simulink model "CF016A_GmVehSpdArbn"  (R2013b)
settings: Solver=FixedStepDiscrete  SolverMode=SingleTasking  StartTime=0.0  StopTime=1  FixedStep=0.002  RelTol=1e-3
undefined symbols (not defined in the file): DIAGCSTRTUPDLY_CNT_U32, NODEBSTEP_CNT_U16, NtcNr1, NtcSts1, VEHSPDMAX_KPH_F32
libraries: simulink x8, NxtrMax x7, NxtrMin x3, NxtrLim x3
(part 1 of 5)
settings Model: PauseTimes=2  CovMetricSettings=dcmrw  CovFilter=CF09_GMOverlayStateHandler_v002_covfilter  CovHTMLOptions=-sRT=1 -aTS=1 -bRG=1 -bTC=1 -hTR=0 -nFC=0 -scm=1 -bcm=1 -xEv=0  covSaveCumulativeToWorkspaceVar=off  CovSaveSingleToWorkspaceVar=off  CovCumulativeReport=on  Creator=SZ7VY6  LastModifiedBy=sz7vy6
settings SolverCC: AutoInsertRateTranBlk=on  InsertRTBMode=Always
settings DataIOCC: LimitDataPoints=off  SaveFormat=Structure  ReturnWorkspaceOutputs=on
settings OptimizationCC: BlockReduction=off  InlineParams=on  ZeroExternalMemoryAtStartup=off  ZeroInternalMemoryAtStartup=off  OptimizeModelRefInitCode=on  LifeSpan=1
settings DebuggingCC: SignalInfNanChecking=error  SignalRangeChecking=warning  UnderspecifiedInitializationDetection=Simplified  SolverPrmCheckMsg=error  InheritedTsInSrcMsg=error  DiscreteInheritContinuousMsg=error  SingleTaskRateTransMsg=error  TasksWithSamePriorityMsg=error  SigSpecEnsureSampleTimeMsg=error  CheckMatrixSingularityMsg=error  ParameterUnderflowMsg=error  ParameterPrecisionLossMsg=error  ParameterTunabilityLossMsg=error  FixptConstUnderflowMsg=warning  FixptConstOverflowMsg=warning  VectorMatrixConversionMsg=error  SignalLabelMismatchMsg=error  UnconnectedInputMsg=error  UnconnectedOutputMsg=error  UnconnectedLineMsg=error  SFcnCompatibilityMsg=error  UniqueDataStoreMsg=warning  BusObjectLabelMismatch=error  RootOutportRequireBusObject=error  AssertControl=DisableAll  ModelReferenceIOMsg=error  ModelReferenceVersionMismatchMessage=warning  ModelReferenceIOMismatchMessage=error  ModelReferenceCSMismatchMessage=warning  ModelReferenceDataLoggingMessage=error  StateNameClashWarn=warning  StrictBusMsg=ErrorOnBusTreatedAsVector  NonBusSignalsTreatedAsBus=error  SFUnexpectedBacktrackingDiag=error  SFInvalidInputDataAccessInChartInitDiag=error  SFNoUnconditionalDefaultTransitionDiag=error  SFTransitionOutsideNaturalParentDiag=error  SFUnconditionalTransitionShadowingDiag=error  SFUndirectedBroadcastEventsDiag=error
settings ModelReferenceCC: ModelReferenceNumInstancesAllowed=Single
settings RTWCC: SystemTargetFile=autosar.tlc  GenCodeOnly=on  TemplateMakefile=ert_default_tmf  Description=AUTOSAR  GenerateReport=on  ProcessScript=autosar_make_rtw_hook  LaunchReport=on
settings CodeAppCC: GenerateComments=off  IgnoreCustomStorageClasses=off  CustomSymbolStrType=$N$R$M  CustomSymbolStrBlkIO=$N$M  SimulinkBlockComments=off
settings STFCustomTargetCC: ParMdlRefBuildCompliant=on  CompOptLevelCompliant=on  IncludeMdlTerminateFcn=off  CombineOutputUpdateFcns=on  SuppressErrorStatus=on  ERTFirstTimeCompliant=on  ERTCustomFileBanners=on  SupportNonFinite=off  SupportComplex=off  SupportContinuousTime=off  SupportNonInlinedSFcns=off  MATLABClassNameForMDSCustomization=Simulink.SoftwareTarget.ERTCustomization  AutosarCompliant=on  GRTInterface=off  SystemTargetFile=autosar.tlc
settings ERTTargetCC: CodeReplacementLibrary=ANSI_C  ConcurrentExecutionCompliant=off  IncludeMdlTerminateFcn=off  SuppressErrorStatus=on  SupportNonFinite=off  SupportComplex=off  ModelStepFunctionPrototypeControlCompliant=off  CPPClassGenCompliant=off  AutosarCompliant=on  InlinedParameterPlacement=NonHierarchical  ERTCustomFileTemplate=example_file_process.tlc  EnableUserReplacementTypes=on

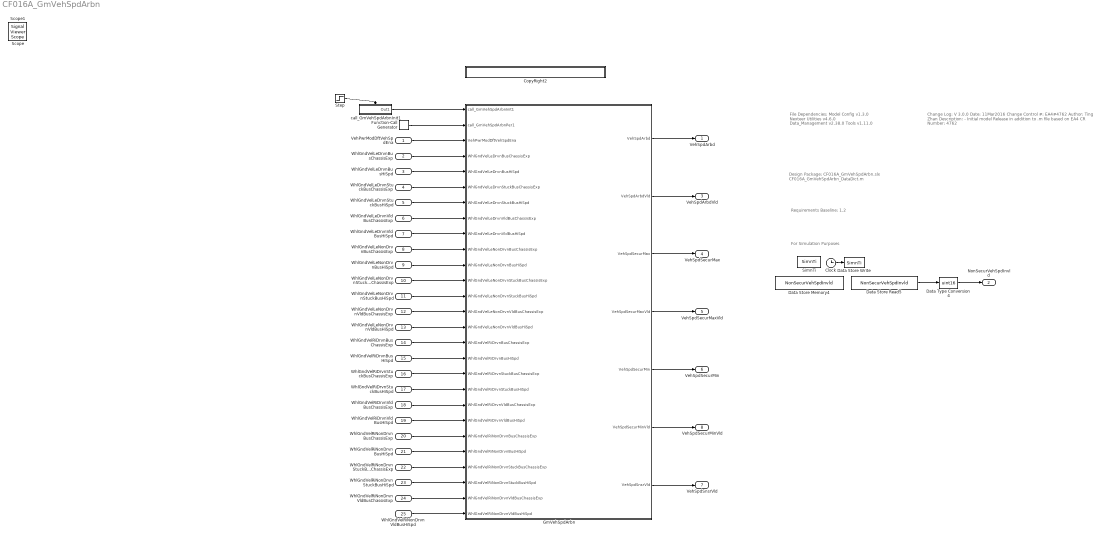
== system CF016A_GmVehSpdArbn ==
  note: File Dependencies:
      |
      | Model Config v1.3.0
      | Nexteer Utilities v4.6.0
      | Data_Management v2.38.0
      | Tools v1.11.0
  note: Requirements Baseline: 1.2
  note: Change Log:
      |
      | V 3.0.0
      | Date: 11Mar2016
      | Change Control #: EA4#4762
      | Author: Ting Zhan
      | Description:
      | - Initial model Release in addition to .m file based on EA4
      | CR Number: 4762
  note: For Simulation Purposes
  note: Design Package:
      | CF016A_GmVehSpdArbn.slx
      | CF016A_GmVehSpdArbn_DataDict.m
  VehPwrModDftVehSpdEna : Inport  RequirementInfo={} %GIDa_1b9c6812_2c02_4b85_9a2c_669458cc48bb  OutDataTypeStr=boolean
  WhlGndVelLeDrvnBusChassisExp : Inport  RequirementInfo={} %GIDa_f6a8d43a_8d7a_4621_b19c_bbf61fc3f1fb  Port=2  OutDataTypeStr=single
  WhlGndVelLeDrvnBusHiSpd : Inport  RequirementInfo={} %GIDa_8d06928a_e9dc_4bb5_bb38_60b41e7e1a37  Port=3  OutDataTypeStr=single
  WhlGndVelLeDrvnStuckBusChassisExp : Inport  RequirementInfo={} %GIDa_37f18a4c_7dd2_4559_8edf_851675215370  Port=4  OutDataTypeStr=boolean
  WhlGndVelLeDrvnStuckBusHiSpd : Inport  RequirementInfo={} %GIDa_387e051a_cae3_4bd1_96b6_4bb2f8da8f18  Port=5  OutDataTypeStr=boolean
  WhlGndVelLeDrvnVldBusChassisExp : Inport  RequirementInfo={} %GIDa_835686fb_41df_4b3b_981b_1312eb084a3e  Port=6  OutDataTypeStr=boolean
  WhlGndVelLeDrvnVldBusHiSpd : Inport  RequirementInfo={} %GIDa_951897dd_207e_4223_8bb8_db091924bf4f  Port=7  OutDataTypeStr=boolean
  WhlGndVelLeNonDrvnBusChassisExp : Inport  RequirementInfo={} %GIDa_a4eac490_54c7_4771_95de_17d76ce0ec27  Port=8  OutDataTypeStr=single
  WhlGndVelLeNonDrvnBusHiSpd : Inport  RequirementInfo={} %GIDa_08a6082e_b874_4a55_b94e_1af7c22679ef  Port=9  OutDataTypeStr=single
  WhlGndVelLeNonDrvnStuckBusChassisExp : Inport  RequirementInfo={} %GIDa_8ce78da2_9eb9_457c_9700_f53d3d0bd86d  Port=10  OutDataTypeStr=boolean
  WhlGndVelLeNonDrvnStuckBusHiSpd : Inport  RequirementInfo={} %GIDa_514e7ca7_7671_44d6_bb21_5a584f285d08  Port=11  OutDataTypeStr=boolean
  WhlGndVelLeNonDrvnVldBusChassisExp : Inport  RequirementInfo={} %GIDa_350e08e4_76f4_4ea8_8a72_cd9a2d5bb9fc  Port=12  OutDataTypeStr=boolean
  WhlGndVelLeNonDrvnVldBusHiSpd : Inport  RequirementInfo={} %GIDa_e452ab69_b19c_414f_baf2_b1cca5193dc7  Port=13  OutDataTypeStr=boolean
  WhlGndVelRiDrvnBusChassisExp : Inport  RequirementInfo={} %GIDa_febb2255_174e_400c_a750_3a2634fb8d82  Port=14  OutDataTypeStr=single
  WhlGndVelRiDrvnBusHiSpd : Inport  RequirementInfo={} %GIDa_33e5a17e_e6ff_4c9b_8e04_aa687b674ac0  Port=15  OutDataTypeStr=single
  WhlGndVelRiDrvnStuckBusChassisExp : Inport  RequirementInfo={} %GIDa_eb4592a4_6e28_4790_a7e9_7dfcd52d8359  Port=16  OutDataTypeStr=boolean
  WhlGndVelRiDrvnStuckBusHiSpd : Inport  RequirementInfo={} %GIDa_4d5fec21_2deb_48fd_8ba8_4b270e8dc755  Port=17  OutDataTypeStr=boolean
  WhlGndVelRiDrvnVldBusChassisExp : Inport  RequirementInfo={} %GIDa_0045e6f2_b2f6_4af3_8c4b_d2a93e5e542f  Port=18  OutDataTypeStr=boolean
  WhlGndVelRiDrvnVldBusHiSpd : Inport  RequirementInfo={} %GIDa_aa92ccdb_2b03_48a5_9a02_c9af57aaf9ac  Port=19  OutDataTypeStr=boolean
  WhlGndVelRiNonDrvnBusChassisExp : Inport  RequirementInfo={} %GIDa_6a49e4d8_e7ef_45b6_ac02_9148e779a1b3  Port=20  OutDataTypeStr=single
  WhlGndVelRiNonDrvnBusHiSpd : Inport  RequirementInfo={} %GIDa_c3dbff61_00f7_4638_9308_f36d29dc0e51  Port=21  OutDataTypeStr=single
  WhlGndVelRiNonDrvnStuckBusChassisExp : Inport  RequirementInfo={} %GIDa_d960e54b_b41b_4df2_9791_080f8c78f146  Port=22  OutDataTypeStr=boolean
  WhlGndVelRiNonDrvnStuckBusHiSpd : Inport  RequirementInfo={} %GIDa_679668c6_3c13_4074_8295_9c18477c1537  Port=23  OutDataTypeStr=boolean
  WhlGndVelRiNonDrvnVldBusChassisExp : Inport  RequirementInfo={} %GIDa_7aefde58_d94c_4a0b_882a_fddc487b4430  Port=24  OutDataTypeStr=boolean
  WhlGndVelRiNonDrvnVldBusHiSpd : Inport  RequirementInfo={} %GIDa_14985695_b713_4ff3_87b9_d780a2a8766e  Port=25  OutDataTypeStr=boolean
  Clock : Clock
  CopyRight2 : Subsystem  Description=|  mask(Copyright Information){none=on}
      | Copyright info block.                                               
      |                                                                     
      | Place copyright information at the top of every subsystem in design.
      mask prompts: none "No parameters"
      mask help: Place copyright information at the top of every subsystem in design.
      mask Display:
      | NxtrConf = 'Nexteer Confidential';
      | 
      | sys = bdroot; %handle for the current model ("system")
      | first = get_param(sys,'Created');
      | if(isempty(first))
      |     first = datestr(now,'yyyy');
      | else
      |     first = first(end-3:end);  %year is last four digits
      | end
      | 
      | last = get_param(sys,'LastModifiedDate');
      | if isempty(last)
      |     last = datestr(now,'yyyy');
      | else
      |     last = last(end-3:end);
      | end
      | 
      | if strcmp(first,last)
      |     fprintf('%s -- Copyright %s Nexteer',NxtrConf,first)
      | else
      |     fprintf('%s -- %s%s- %s Nexteer',NxtrConf,char(169),first,last)
      | end
  Data Store Memory4 : DataStoreMemory  DataStoreName=NonSecurVehSpdInvld  InitialValue=NtcSts1.NTCSTS_PASSD  OutDataTypeStr=Enum: NtcSts1
  Data Store Read5 : DataStoreRead  DataStoreName=NonSecurVehSpdInvld  SampleTime=.004
  Data Store Write : DataStoreWrite  DataStoreName=SimnTi
  Data Type Conversion4 : DataTypeConversion  OutDataTypeStr=uint16
  Function-Call Generator : simulink/Ports & Subsystems/Function-Call Generator  sample_time=.01  numberOfIterations=1
      settings: AttributesFormatString=%<sample_time>
  GmVehSpdArbn : Subsystem  RequirementInfo="{}  %GIDa_c04c64db_09f4_4bf6_ae81_75ae0555dc21"
  SimnTi : DataStoreMemory  DataStoreName=SimnTi
  Step : Step  Time=.001  Before=1  After=0  SampleTime=0
  call_GmVehSpdArbnInit1 : Subsystem  TreatAsAtomicUnit=on
  VehSpdArbd : Outport  RequirementInfo={} %GIDa_1da87020_2114_47f8_bd6a_dcf122c70ef9
  NonSecurVehSpdInvld : Outport  RequirementInfo={} %GIDa_f8f24313_b0b7_4842_bede_f0c570d36cae  Port=2
  VehSpdArbdVld : Outport  RequirementInfo={} %GIDa_aeae8495_df44_455f_bfcb_3785565b89f3  Port=3
  VehSpdSecurMax : Outport  RequirementInfo={} %GIDa_e60aac24_3e4f_4fa4_92d1_30c110927cae  Port=4
  VehSpdSecurMaxVld : Outport  RequirementInfo={} %GIDa_e0614fd2_7d45_427f_a7be_e9487d2cc3f6  Port=5
  VehSpdSecurMin : Outport  RequirementInfo={} %GIDa_5226fce9_09b3_4eff_a0f8_954e16115eec  Port=6
  VehSpdSnsrVld : Outport  RequirementInfo={} %GIDa_37fde451_082a_4d0c_b5e1_d1c1d8bf7c50  Port=7
  VehSpdSecurMinVld : Outport  RequirementInfo={} %GIDa_3de6a7fd_89af_4cb9_baa0_fb7c34e7cace  Port=8
  Scope : SignalViewerScope  IOType=viewer  RefreshTime=0.035000
  Scope1 : SignalViewerScope  IOType=viewer  RefreshTime=0.035000
  wires:
  Step/1 -> call_GmVehSpdArbnInit1/Enable
  call_GmVehSpdArbnInit1/1(Out1) -> GmVehSpdArbn/1(call_GmVehSpdArbnInit1)
  Clock/1 -> Data Store Write/1
  GmVehSpdArbn/1(VehSpdArbd) -> VehSpdArbd/1
  Data Store Read5/1 -> Data Type Conversion4/1
  Data Type Conversion4/1 -> NonSecurVehSpdInvld/1
  Function-Call Generator/1 -> GmVehSpdArbn/2(call_GmVehSpdArbnPer1)
  VehPwrModDftVehSpdEna/1 -> GmVehSpdArbn/3(VehPwrModDftVehSpdEna)
  WhlGndVelLeDrvnBusChassisExp/1 -> GmVehSpdArbn/4(WhlGndVelLeDrvnBusChassisExp)
  WhlGndVelLeDrvnBusHiSpd/1 -> GmVehSpdArbn/5(WhlGndVelLeDrvnBusHiSpd)
  WhlGndVelLeDrvnStuckBusChassisExp/1 -> GmVehSpdArbn/6(WhlGndVelLeDrvnStuckBusChassisExp)
  WhlGndVelLeDrvnStuckBusHiSpd/1 -> GmVehSpdArbn/7(WhlGndVelLeDrvnStuckBusHiSpd)
  WhlGndVelLeDrvnVldBusChassisExp/1 -> GmVehSpdArbn/8(WhlGndVelLeDrvnVldBusChassisExp)
  WhlGndVelLeDrvnVldBusHiSpd/1 -> GmVehSpdArbn/9(WhlGndVelLeDrvnVldBusHiSpd)
  WhlGndVelLeNonDrvnBusChassisExp/1 -> GmVehSpdArbn/10(WhlGndVelLeNonDrvnBusChassisExp)
  WhlGndVelLeNonDrvnBusHiSpd/1 -> GmVehSpdArbn/11(WhlGndVelLeNonDrvnBusHiSpd)
  WhlGndVelLeNonDrvnStuckBusChassisExp/1 -> GmVehSpdArbn/12(WhlGndVelLeNonDrvnStuckBusChassisExp)
  WhlGndVelLeNonDrvnStuckBusHiSpd/1 -> GmVehSpdArbn/13(WhlGndVelLeNonDrvnStuckBusHiSpd)
  WhlGndVelLeNonDrvnVldBusChassisExp/1 -> GmVehSpdArbn/14(WhlGndVelLeNonDrvnVldBusChassisExp)
  WhlGndVelLeNonDrvnVldBusHiSpd/1 -> GmVehSpdArbn/15(WhlGndVelLeNonDrvnVldBusHiSpd)
  WhlGndVelRiDrvnBusChassisExp/1 -> GmVehSpdArbn/16(WhlGndVelRiDrvnBusChassisExp)
  WhlGndVelRiDrvnBusHiSpd/1 -> GmVehSpdArbn/17(WhlGndVelRiDrvnBusHiSpd)
  WhlGndVelRiDrvnStuckBusChassisExp/1 -> GmVehSpdArbn/18(WhlGndVelRiDrvnStuckBusChassisExp)
  WhlGndVelRiDrvnStuckBusHiSpd/1 -> GmVehSpdArbn/19(WhlGndVelRiDrvnStuckBusHiSpd)
  WhlGndVelRiDrvnVldBusChassisExp/1 -> GmVehSpdArbn/20(WhlGndVelRiDrvnVldBusChassisExp)
  WhlGndVelRiDrvnVldBusHiSpd/1 -> GmVehSpdArbn/21(WhlGndVelRiDrvnVldBusHiSpd)
  WhlGndVelRiNonDrvnBusChassisExp/1 -> GmVehSpdArbn/22(WhlGndVelRiNonDrvnBusChassisExp)
  WhlGndVelRiNonDrvnBusHiSpd/1 -> GmVehSpdArbn/23(WhlGndVelRiNonDrvnBusHiSpd)
  WhlGndVelRiNonDrvnStuckBusChassisExp/1 -> GmVehSpdArbn/24(WhlGndVelRiNonDrvnStuckBusChassisExp)
  WhlGndVelRiNonDrvnStuckBusHiSpd/1 -> GmVehSpdArbn/25(WhlGndVelRiNonDrvnStuckBusHiSpd)
  WhlGndVelRiNonDrvnVldBusChassisExp/1 -> GmVehSpdArbn/26(WhlGndVelRiNonDrvnVldBusChassisExp)
  WhlGndVelRiNonDrvnVldBusHiSpd/1 -> GmVehSpdArbn/27(WhlGndVelRiNonDrvnVldBusHiSpd)
  GmVehSpdArbn/2(VehSpdArbdVld) -> VehSpdArbdVld/1
  GmVehSpdArbn/7(VehSpdSnsrVld) -> VehSpdSnsrVld/1
  GmVehSpdArbn/3(VehSpdSecurMax) -> VehSpdSecurMax/1
  GmVehSpdArbn/4(VehSpdSecurMaxVld) -> VehSpdSecurMaxVld/1
  GmVehSpdArbn/5(VehSpdSecurMin) -> VehSpdSecurMin/1
  GmVehSpdArbn/6(VehSpdSecurMinVld) -> VehSpdSecurMinVld/1

== system CF016A_GmVehSpdArbn/CopyRight2 ==

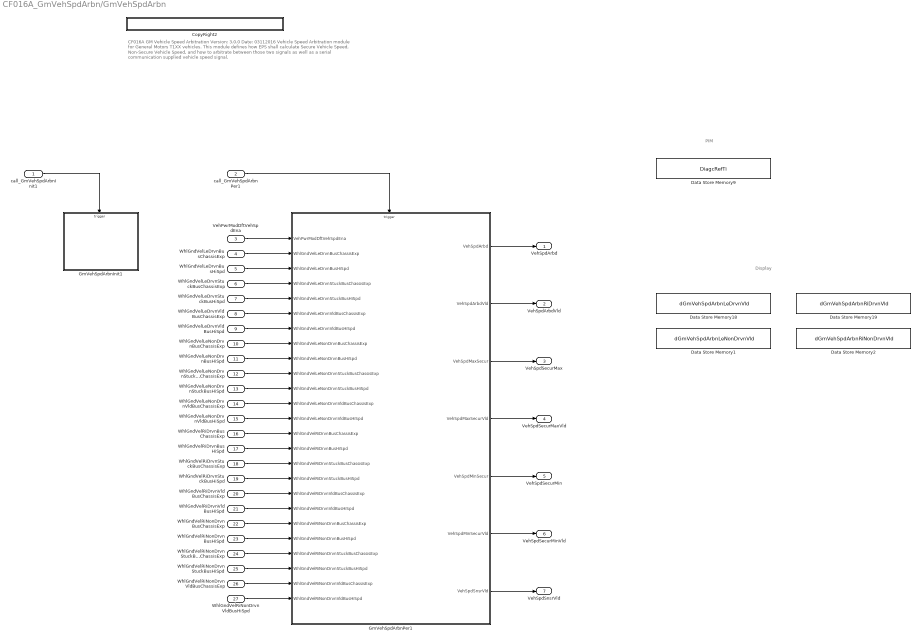
== system CF016A_GmVehSpdArbn/GmVehSpdArbn ==
  note: CF016A  GM Vehicle Speed Arbitration
      | Version: 3.0.0      Date: 03112016
      |
      | Vehicle Speed Arbitration module for General Motors T1XX vehicles. This module defines how EPS shall calculate Secure Vehicle Speed, Non-Secure Vehicle Speed,
      | and how to arbitrate between those two signals as well as a serial communication supplied vehicle speed signal.
  note: PIM
  note: Display
  call_GmVehSpdArbnInit1 : Inport  RequirementInfo={} %GIDa_bfdeb5c8_34d3_4847_8322_14533b8a1ec7
  call_GmVehSpdArbnPer1 : Inport  RequirementInfo={} %GIDa_f1c70cb1_f5af_488b_94e7_678758a8a022  Port=2
  VehPwrModDftVehSpdEna : Inport  RequirementInfo="{'linktype_rmi_doors' '0000c6e6 (/GM T1XX/SubSystem Specifications/Customer Functions/CF016A GM Vehicle Speed Arbitration)' '#202' 'true' 'REQ:  202' '' } %GIDa_dae255f8_68ff_4c98_b110_bcea0aba3add"  Port=3  OutDataTypeStr=boolean
  WhlGndVelLeDrvnBusChassisExp : Inport  RequirementInfo="{'linktype_rmi_doors' '0000c6e6 (/GM T1XX/SubSystem Specifications/Customer Functions/CF016A GM Vehicle Speed Arbitration)' '#115' 'true' 'REQ:  115' '' } %GIDa_f94e4f25_dea2_4ca1_8f0e_cbc76f57a275"  Port=4  OutDataTypeStr=single
  WhlGndVelLeDrvnBusHiSpd : Inport  RequirementInfo="{'linktype_rmi_doors' '0000c6e6 (/GM T1XX/SubSystem Specifications/Customer Functions/CF016A GM Vehicle Speed Arbitration)' '#107' 'true' 'REQ:  107' '' } %GIDa_669e5e04_64c9_4eb9_af64_7f0439853a42"  Port=5  OutDataTypeStr=single
  WhlGndVelLeDrvnStuckBusChassisExp : Inport  RequirementInfo="{'linktype_rmi_doors' '0000c6e6 (/GM T1XX/SubSystem Specifications/Customer Functions/CF016A GM Vehicle Speed Arbitration)' '#207' 'true' 'REQ:  207' '' } %GIDa_30a67b8a_f2de_4c81_bdbc_3e51fc1fd2c1"  Port=6  OutDataTypeStr=boolean
  WhlGndVelLeDrvnStuckBusHiSpd : Inport  RequirementInfo="{'linktype_rmi_doors' '0000c6e6 (/GM T1XX/SubSystem Specifications/Customer Functions/CF016A GM Vehicle Speed Arbitration)' '#211' 'true' 'REQ:  211' '' } %GIDa_2439a840_dfd0_4d26_afae_da33f00f7dcf"  Port=7  OutDataTypeStr=boolean
  WhlGndVelLeDrvnVldBusChassisExp : Inport  RequirementInfo="{'linktype_rmi_doors' '0000c6e6 (/GM T1XX/SubSystem Specifications/Customer Functions/CF016A GM Vehicle Speed Arbitration)' '#110' 'true' 'REQ:  110' '' } %GIDa_e405ee3d_6faa_40e1_bd85_7a185fe78396"  Port=8  OutDataTypeStr=boolean
  WhlGndVelLeDrvnVldBusHiSpd : Inport  RequirementInfo="{'linktype_rmi_doors' '0000c6e6 (/GM T1XX/SubSystem Specifications/Customer Functions/CF016A GM Vehicle Speed Arbitration)' '#43' 'true' 'REQ:  43' '' } %GIDa_12c1b163_feda_400f_9b5a_3f16f6c62cf6"  Port=9  OutDataTypeStr=boolean
  WhlGndVelLeNonDrvnBusChassisExp : Inport  RequirementInfo="{'linktype_rmi_doors' '0000c6e6 (/GM T1XX/SubSystem Specifications/Customer Functions/CF016A GM Vehicle Speed Arbitration)' '#119' 'true' 'REQ:  119' '' } %GIDa_39e72722_187f_45b0_998e_09f5390847cd"  Port=10  OutDataTypeStr=single
  WhlGndVelLeNonDrvnBusHiSpd : Inport  RequirementInfo="{'linktype_rmi_doors' '0000c6e6 (/GM T1XX/SubSystem Specifications/Customer Functions/CF016A GM Vehicle Speed Arbitration)' '#116' 'true' 'REQ:  116' '' } %GIDa_97eaef5a_2083_4cc9_9391_474d7ce2a873"  Port=11  OutDataTypeStr=single
  WhlGndVelLeNonDrvnStuckBusChassisExp : Inport  RequirementInfo="{'linktype_rmi_doors' '0000c6e6 (/GM T1XX/SubSystem Specifications/Customer Functions/CF016A GM Vehicle Speed Arbitration)' '#214' 'true' 'REQ:  214' '' } %GIDa_3774bdb3_ce3e_44e7_ac99_5715957e9824"  Port=12  OutDataTypeStr=boolean
  WhlGndVelLeNonDrvnStuckBusHiSpd : Inport  RequirementInfo="{'linktype_rmi_doors' '0000c6e6 (/GM T1XX/SubSystem Specifications/Customer Functions/CF016A GM Vehicle Speed Arbitration)' '#210' 'true' 'REQ:  210' '' } %GIDa_bed02905_1f15_4bbf_93cd_075107bd0ea2"  Port=13  OutDataTypeStr=boolean
  WhlGndVelLeNonDrvnVldBusChassisExp : Inport  RequirementInfo="{'linktype_rmi_doors' '0000c6e6 (/GM T1XX/SubSystem Specifications/Customer Functions/CF016A GM Vehicle Speed Arbitration)' '#112' 'true' 'REQ:  112' '' } %GIDa_d30fd230_2b58_41b0_a7f1_e482c8502763"  Port=14  OutDataTypeStr=boolean
  WhlGndVelLeNonDrvnVldBusHiSpd : Inport  RequirementInfo="{'linktype_rmi_doors' '0000c6e6 (/GM T1XX/SubSystem Specifications/Customer Functions/CF016A GM Vehicle Speed Arbitration)' '#108' 'true' 'REQ:  108' '' } %GIDa_4eae57c8_8600_40ef_b8ac_9b189ac57f7a"  Port=15  OutDataTypeStr=boolean
  WhlGndVelRiDrvnBusChassisExp : Inport  RequirementInfo="{'linktype_rmi_doors' '0000c6e6 (/GM T1XX/SubSystem Specifications/Customer Functions/CF016A GM Vehicle Speed Arbitration)' '#114' 'true' 'REQ:  114' '' } %GIDa_6bd502cf_b064_4897_9777_7f6636a1c34f"  Port=16  OutDataTypeStr=single
  WhlGndVelRiDrvnBusHiSpd : Inport  RequirementInfo="{'linktype_rmi_doors' '0000c6e6 (/GM T1XX/SubSystem Specifications/Customer Functions/CF016A GM Vehicle Speed Arbitration)' '#118' 'true' 'REQ:  118' '' } %GIDa_c603ff0a_f493_4b44_bcd9_68a71796a871"  Port=17  OutDataTypeStr=single
  WhlGndVelRiDrvnStuckBusChassisExp : Inport  RequirementInfo="{'linktype_rmi_doors' '0000c6e6 (/GM T1XX/SubSystem Specifications/Customer Functions/CF016A GM Vehicle Speed Arbitration)' '#213' 'true' 'REQ:  213' '' } %GIDa_0f48a0b2_2e47_4a31_bdfc_59f5e7754cf7"  Port=18  OutDataTypeStr=boolean
  WhlGndVelRiDrvnStuckBusHiSpd : Inport  RequirementInfo="{'linktype_rmi_doors' '0000c6e6 (/GM T1XX/SubSystem Specifications/Customer Functions/CF016A GM Vehicle Speed Arbitration)' '#209' 'true' 'REQ:  209' '' } %GIDa_84960805_71e5_496f_bbda_4f40d111b122"  Port=19  OutDataTypeStr=boolean
  WhlGndVelRiDrvnVldBusChassisExp : Inport  RequirementInfo="{'linktype_rmi_doors' '0000c6e6 (/GM T1XX/SubSystem Specifications/Customer Functions/CF016A GM Vehicle Speed Arbitration)' '#111' 'true' 'REQ:  111' '' } %GIDa_dda09a8d_a2b5_4204_b82c_e64290a9a1b3"  Port=20  OutDataTypeStr=boolean
  WhlGndVelRiDrvnVldBusHiSpd : Inport  RequirementInfo="{'linktype_rmi_doors' '0000c6e6 (/GM T1XX/SubSystem Specifications/Customer Functions/CF016A GM Vehicle Speed Arbitration)' '#42' 'true' 'REQ:  42' '' } %GIDa_4fb6dacd_a67a_4808_9647_506e322e7f6f"  Port=21  OutDataTypeStr=boolean
  WhlGndVelRiNonDrvnBusChassisExp : Inport  RequirementInfo="{'linktype_rmi_doors' '0000c6e6 (/GM T1XX/SubSystem Specifications/Customer Functions/CF016A GM Vehicle Speed Arbitration)' '#120' 'true' 'REQ:  120' '' } %GIDa_52ed85e9_1e6a_4f85_9de5_a437e8780bfc"  Port=22  OutDataTypeStr=single
  WhlGndVelRiNonDrvnBusHiSpd : Inport  RequirementInfo="{'linktype_rmi_doors' '0000c6e6 (/GM T1XX/SubSystem Specifications/Customer Functions/CF016A GM Vehicle Speed Arbitration)' '#117' 'true' 'REQ:  117' '' } %GIDa_8f83058a_23a6_4c83_8450_8359a591ebaa"  Port=23  OutDataTypeStr=single
  WhlGndVelRiNonDrvnStuckBusChassisExp : Inport  RequirementInfo="{'linktype_rmi_doors' '0000c6e6 (/GM T1XX/SubSystem Specifications/Customer Functions/CF016A GM Vehicle Speed Arbitration)' '#212' 'true' 'REQ:  212' '' } %GIDa_71e2d22e_b40d_49e2_a3c2_e216d7d1aec1"  Port=24  OutDataTypeStr=boolean
  WhlGndVelRiNonDrvnStuckBusHiSpd : Inport  RequirementInfo="{'linktype_rmi_doors' '0000c6e6 (/GM T1XX/SubSystem Specifications/Customer Functions/CF016A GM Vehicle Speed Arbitration)' '#208' 'true' 'REQ:  208' '' } %GIDa_03ea0a8c_e16c_4679_8a1e_c2428d8348ad"  Port=25  OutDataTypeStr=boolean
  WhlGndVelRiNonDrvnVldBusChassisExp : Inport  RequirementInfo="{'linktype_rmi_doors' '0000c6e6 (/GM T1XX/SubSystem Specifications/Customer Functions/CF016A GM Vehicle Speed Arbitration)' '#113' 'true' 'REQ:  113' '' } %GIDa_07e6057e_bc3a_428f_8ca3_00e8b15c143c"  Port=26  OutDataTypeStr=boolean
  WhlGndVelRiNonDrvnVldBusHiSpd : Inport  RequirementInfo="{'linktype_rmi_doors' '0000c6e6 (/GM T1XX/SubSystem Specifications/Customer Functions/CF016A GM Vehicle Speed Arbitration)' '#109' 'true' 'REQ:  109' '' } %GIDa_20f0f614_c616_4468_aa1a_d68a7b793276"  Port=27  OutDataTypeStr=boolean
  CopyRight2 : Subsystem  Description=|  mask(Copyright Information){none=on}
      | Copyright info block.                                               
      |                                                                     
      | Place copyright information at the top of every subsystem in design.
      mask prompts: none "No parameters"
      mask help: Place copyright information at the top of every subsystem in design.
      mask Display:
      | NxtrConf = 'Nexteer Confidential';
      | 
      | sys = bdroot; %handle for the current model ("system")
      | first = get_param(sys,'Created');
      | if(isempty(first))
      |     first = datestr(now,'yyyy');
      | else
      |     first = first(end-3:end);  %year is last four digits
      | end
      | 
      | last = get_param(sys,'LastModifiedDate');
      | if isempty(last)
      |     last = datestr(now,'yyyy');
      | else
      |     last = last(end-3:end);
      | end
      | 
      | if strcmp(first,last)
      |     fprintf('%s -- Copyright %s Nexteer',NxtrConf,first)
      | else
      |     fprintf('%s -- %s%s- %s Nexteer',NxtrConf,char(169),first,last)
      | end
  Data Store Memory1 : DataStoreMemory  RequirementInfo="{}  %GIDa_1ec8dfb0_664c_42a7_8b07_c6d541348300"  DataStoreName=dGmVehSpdArbnLeNonDrvnVld  StateMustResolveToSignalObject=on
  Data Store Memory18 : DataStoreMemory  RequirementInfo="{}  %GIDa_dccf1f98_b206_44ee_976e_804b06016ae4"  DataStoreName=dGmVehSpdArbnLeDrvnVld  StateMustResolveToSignalObject=on
  Data Store Memory19 : DataStoreMemory  RequirementInfo="{}  %GIDa_fdf38b69_a9a6_40a3_8b2a_5331053cf772"  DataStoreName=dGmVehSpdArbnRiDrvnVld  StateMustResolveToSignalObject=on
  Data Store Memory2 : DataStoreMemory  RequirementInfo="{}  %GIDa_78a29301_78b6_4b65_8bc2_c82305c40bcd"  DataStoreName=dGmVehSpdArbnRiNonDrvnVld  StateMustResolveToSignalObject=on
  Data Store Memory9 : DataStoreMemory  DataStoreName=DiagcRefTi  StateMustResolveToSignalObject=on
  GmVehSpdArbnInit1 : Subsystem
  GmVehSpdArbnPer1 : Subsystem
  VehSpdArbd : Outport  RequirementInfo="{'linktype_rmi_doors' '0000c6e6 (/GM T1XX/SubSystem Specifications/Customer Functions/CF016A GM Vehicle Speed Arbitration)' '#106' 'true' 'REQ:  106' '' } %GIDa_69b1c859_cbd1_4f7d_b737_cd6829536f82"
  VehSpdArbdVld : Outport  RequirementInfo="{'linktype_rmi_doors' '0000c6e6 (/GM T1XX/SubSystem Specifications/Customer Functions/CF016A GM Vehicle Speed Arbitration)' '#186' 'true' 'REQ:  186' '' } %GIDa_7ca0a8c8_fd69_404b_8532_00ddb208e376"  Port=2
  VehSpdSecurMax : Outport  RequirementInfo="{'linktype_rmi_doors' '0000c6e6 (/GM T1XX/SubSystem Specifications/Customer Functions/CF016A GM Vehicle Speed Arbitration)' '#152' 'true' 'REQ:  152' '' } %GIDa_b6124501_08bf_46ef_9740_e78f18fd7388"  Port=3
  VehSpdSecurMaxVld : Outport  RequirementInfo="{'linktype_rmi_doors' '0000c6e6 (/GM T1XX/SubSystem Specifications/Customer Functions/CF016A GM Vehicle Speed Arbitration)' '#189' 'true' 'REQ:  189' '' } %GIDa_863bbd51_b659_47ae_b395_70cee02ee7e0"  Port=4
  VehSpdSecurMin : Outport  RequirementInfo="{'linktype_rmi_doors' '0000c6e6 (/GM T1XX/SubSystem Specifications/Customer Functions/CF016A GM Vehicle Speed Arbitration)' '#153' 'true' 'REQ:  153' '' } %GIDa_8c828841_653f_4def_a75f_5795471f1337"  Port=5
  VehSpdSecurMinVld : Outport  RequirementInfo="{'linktype_rmi_doors' '0000c6e6 (/GM T1XX/SubSystem Specifications/Customer Functions/CF016A GM Vehicle Speed Arbitration)' '#190' 'true' 'REQ:  190' '' } %GIDa_b8287d43_1a15_44b1_94d7_53b3f5775143"  Port=6
  VehSpdSnsrVld : Outport  RequirementInfo="{'linktype_rmi_doors' '0000c6e6 (/GM T1XX/SubSystem Specifications/Customer Functions/CF016A GM Vehicle Speed Arbitration)' '#222' 'true' 'REQ:  222' '' } %GIDa_b2111448_4c03_44d3_a274_c2c7a4d7a68d"  Port=7
  wires:
  call_GmVehSpdArbnPer1/1 -> GmVehSpdArbnPer1/Trigger
  call_GmVehSpdArbnInit1/1 -> GmVehSpdArbnInit1/Trigger
  VehPwrModDftVehSpdEna/1 -> GmVehSpdArbnPer1/1(VehPwrModDftVehSpdEna)
  WhlGndVelLeDrvnBusChassisExp/1 -> GmVehSpdArbnPer1/2(WhlGndVelLeDrvnBusChassisExp)
  WhlGndVelLeDrvnBusHiSpd/1 -> GmVehSpdArbnPer1/3(WhlGndVelLeDrvnBusHiSpd)
  WhlGndVelLeDrvnStuckBusChassisExp/1 -> GmVehSpdArbnPer1/4(WhlGndVelLeDrvnStuckBusChassisExp)
  WhlGndVelLeDrvnStuckBusHiSpd/1 -> GmVehSpdArbnPer1/5(WhlGndVelLeDrvnStuckBusHiSpd)
  WhlGndVelLeDrvnVldBusChassisExp/1 -> GmVehSpdArbnPer1/6(WhlGndVelLeDrvnVldBusChassisExp)
  WhlGndVelLeDrvnVldBusHiSpd/1 -> GmVehSpdArbnPer1/7(WhlGndVelLeDrvnVldBusHiSpd)
  WhlGndVelLeNonDrvnBusChassisExp/1 -> GmVehSpdArbnPer1/8(WhlGndVelLeNonDrvnBusChassisExp)
  WhlGndVelLeNonDrvnBusHiSpd/1 -> GmVehSpdArbnPer1/9(WhlGndVelLeNonDrvnBusHiSpd)
  WhlGndVelLeNonDrvnStuckBusChassisExp/1 -> GmVehSpdArbnPer1/10(WhlGndVelLeNonDrvnStuckBusChassisExp)
  WhlGndVelLeNonDrvnStuckBusHiSpd/1 -> GmVehSpdArbnPer1/11(WhlGndVelLeNonDrvnStuckBusHiSpd)
  WhlGndVelLeNonDrvnVldBusChassisExp/1 -> GmVehSpdArbnPer1/12(WhlGndVelLeNonDrvnVldBusChassisExp)
  WhlGndVelLeNonDrvnVldBusHiSpd/1 -> GmVehSpdArbnPer1/13(WhlGndVelLeNonDrvnVldBusHiSpd)
  WhlGndVelRiDrvnBusChassisExp/1 -> GmVehSpdArbnPer1/14(WhlGndVelRiDrvnBusChassisExp)
  WhlGndVelRiDrvnBusHiSpd/1 -> GmVehSpdArbnPer1/15(WhlGndVelRiDrvnBusHiSpd)
  WhlGndVelRiDrvnStuckBusChassisExp/1 -> GmVehSpdArbnPer1/16(WhlGndVelRiDrvnStuckBusChassisExp)
  WhlGndVelRiDrvnStuckBusHiSpd/1 -> GmVehSpdArbnPer1/17(WhlGndVelRiDrvnStuckBusHiSpd)
  WhlGndVelRiDrvnVldBusChassisExp/1 -> GmVehSpdArbnPer1/18(WhlGndVelRiDrvnVldBusChassisExp)
  WhlGndVelRiDrvnVldBusHiSpd/1 -> GmVehSpdArbnPer1/19(WhlGndVelRiDrvnVldBusHiSpd)
  WhlGndVelRiNonDrvnBusChassisExp/1 -> GmVehSpdArbnPer1/20(WhlGndVelRiNonDrvnBusChassisExp)
  WhlGndVelRiNonDrvnBusHiSpd/1 -> GmVehSpdArbnPer1/21(WhlGndVelRiNonDrvnBusHiSpd)
  WhlGndVelRiNonDrvnStuckBusChassisExp/1 -> GmVehSpdArbnPer1/22(WhlGndVelRiNonDrvnStuckBusChassisExp)
  WhlGndVelRiNonDrvnStuckBusHiSpd/1 -> GmVehSpdArbnPer1/23(WhlGndVelRiNonDrvnStuckBusHiSpd)
  WhlGndVelRiNonDrvnVldBusChassisExp/1 -> GmVehSpdArbnPer1/24(WhlGndVelRiNonDrvnVldBusChassisExp)
  WhlGndVelRiNonDrvnVldBusHiSpd/1 -> GmVehSpdArbnPer1/25(WhlGndVelRiNonDrvnVldBusHiSpd)
  GmVehSpdArbnPer1/1(VehSpdArbd) -> VehSpdArbd/1
  GmVehSpdArbnPer1/2(VehSpdArbdVld) -> VehSpdArbdVld/1
  GmVehSpdArbnPer1/7(VehSpdSnsrVld) -> VehSpdSnsrVld/1
  GmVehSpdArbnPer1/3(VehSpdMaxSecur) -> VehSpdSecurMax/1
  GmVehSpdArbnPer1/4(VehSpdMaxSecurVld) -> VehSpdSecurMaxVld/1
  GmVehSpdArbnPer1/5(VehSpdMinSecur) -> VehSpdSecurMin/1
  GmVehSpdArbnPer1/6(VehSpdMinSecurVld) -> VehSpdSecurMinVld/1

== system CF016A_GmVehSpdArbn/call_GmVehSpdArbnInit1 ==
  Enable : EnablePort
  CopyRight2 : Subsystem  Description=|  mask(Copyright Information){none=on}
      | Copyright info block.                                               
      |                                                                     
      | Place copyright information at the top of every subsystem in design.
      mask prompts: none "No parameters"
      mask help: Place copyright information at the top of every subsystem in design.
      mask Display:
      | NxtrConf = 'Nexteer Confidential';
      | 
      | sys = bdroot; %handle for the current model ("system")
      | first = get_param(sys,'Created');
      | if(isempty(first))
      |     first = datestr(now,'yyyy');
      | else
      |     first = first(end-3:end);  %year is last four digits
      | end
      | 
      | last = get_param(sys,'LastModifiedDate');
      | if isempty(last)
      |     last = datestr(now,'yyyy');
      | else
      |     last = last(end-3:end);
      | end
      | 
      | if strcmp(first,last)
      |     fprintf('%s -- Copyright %s Nexteer',NxtrConf,first)
      | else
      |     fprintf('%s -- %s%s- %s Nexteer',NxtrConf,char(169),first,last)
      | end
  call_GmVehSpdArbnInit1 : simulink/Ports & Subsystems/Function-Call Generator  sample_time=.002  numberOfIterations=1
  Out1 : Outport
  wires:
  call_GmVehSpdArbnInit1/1 -> Out1/1

== system CF016A_GmVehSpdArbn/GmVehSpdArbn/CopyRight2 ==

== system CF016A_GmVehSpdArbn/GmVehSpdArbn/GmVehSpdArbnInit1 ==
  function : TriggerPort  TriggerType=function-call
  CopyRight2 : Subsystem  Description=|  mask(Copyright Information){none=on}
      | Copyright info block.                                               
      |                                                                     
      | Place copyright information at the top of every subsystem in design.
      mask prompts: none "No parameters"
      mask help: Place copyright information at the top of every subsystem in design.
      mask Display:
      | NxtrConf = 'Nexteer Confidential';
      | 
      | sys = bdroot; %handle for the current model ("system")
      | first = get_param(sys,'Created');
      | if(isempty(first))
      |     first = datestr(now,'yyyy');
      | else
      |     first = first(end-3:end);  %year is last four digits
      | end
      | 
      | last = get_param(sys,'LastModifiedDate');
      | if isempty(last)
      |     last = datestr(now,'yyyy');
      | else
      |     last = last(end-3:end);
      | end
      | 
      | if strcmp(first,last)
      |     fprintf('%s -- Copyright %s Nexteer',NxtrConf,first)
      | else
      |     fprintf('%s -- %s%s- %s Nexteer',NxtrConf,char(169),first,last)
      | end
  Data Store Write1 : DataStoreWrite  DataStoreName=DiagcRefTi
      settings: AttributesFormatString=%<Priority>
  GetRefTmr100MicroSec32bit : Subsystem
  wires:
  GetRefTmr100MicroSec32bit/1(RefTmr) -> Data Store Write1/1
